simulink model "TX_Model"  (R2017a)
settings: Solver=VariableStepDiscrete  StartTime=0.0  StopTime=0.01  FixedStep=1/(PSF_SampPerSym*Rsymbol*2)  RelTol=1e-3  EnableMultiTasking=on
PreLoadFcn:
  | %Rates
  | BitRate=250e3;
  | ChipRate=2e6;
  | SymRate=ChipRate/2;
  | RX_ChipDelay=6;
  | 
  | 
  | %Pulse shaping filter
  | OS=32;
  | 
  | %Input Power
  | Pin=-12;
InitFcn:
  | x=linspace(0,1,OS);
  | weights=sin(pi*x);
libraries: dspmlti4 x1, commrandsrc2 x1, commseqgen2 x1, dspmathops x1, commdigbbndpm3 x1
settings Model: Creator=The MathWorks Inc.  LastModifiedBy=gzucchel
settings DataIOCC: LimitDataPoints=on  SaveFormat=Array  SignalLoggingSaveFormat=ModelDataLogs  SaveOutput=off  SignalLogging=off  DSMLogging=off  SaveTime=off
settings OptimizationCC: ExpressionDepthLimit=2147483647  LifeSpan=inf
settings DebuggingCC: UnderspecifiedInitializationDetection=Classic  MergeDetectMultiDrivingBlocksExec=none  SolverPrmCheckMsg=warning  FcnCallInpInsideContextMsg=warning  StateNameClashWarn=warning  SFUnexpectedBacktrackingDiag=warning  SFNoUnconditionalDefaultTransitionDiag=warning  SFExecutionAtInitializationDiag=none
settings HardwareCC: ProdBitPerPointer=32  ProdBitPerSizeT=32  ProdBitPerPtrDiffT=32  ProdLargestAtomicFloat=None  ProdIntDivRoundTo=Undefined  ProdEndianess=Unspecified  ProdWordSize=32  ProdHWDeviceType=32-bit Generic
settings ModelReferenceCC: PropagateSignalLabelsOutOfModel=off
settings GRTTargetCC: TargetLangStandard=C89/C90 (ANSI)  GeneratePreprocessorConditionals=Disable all  CombineOutputUpdateFcns=off  GRTInterface=on
settings ConfigComp: CovMetricSettings=dw  CovHtmlReporting=on  CovSaveCumulativeToWorkspaceVar=on  CovSaveSingleToWorkspaceVar=on  CovExternalEMLEnable=off  CovSFcnEnable=off
settings SimscapeCC: SimscapeNormalizeSystem=off  SimscapeNominalValues="[{\"value\":\"10\",\"unit\":\"V\"},{\"value\":\"1\",\"unit\":\"A\"},{\"value\":\"10\",\"unit\":\"N*m\"},{\"value\":\"10\",\"unit\":\"bar\"},{\"value\":\"100\",\"unit\":\"kJ/kg\"},{\"value\":\"1\",\"unit\":\"kW\"},{\"value\":\"300\",\"unit\":\"K\"},{\"value\":\"100\",\"unit\":\"cm^3/s\"},{\"value\":\"1\",\"unit\":\"kN\"},{\"value\":\"1\",\"unit\":\"g/cm^3\"},{\"value\":\"1\",\"unit\":\"l\"},{\"value\":\"1\",\"unit\":\"cm^2\"},{\"value\":\"60\",\"unit\":\"Hz\"}]"
settings ConfigurationSet: Description=SimMechanics 2G

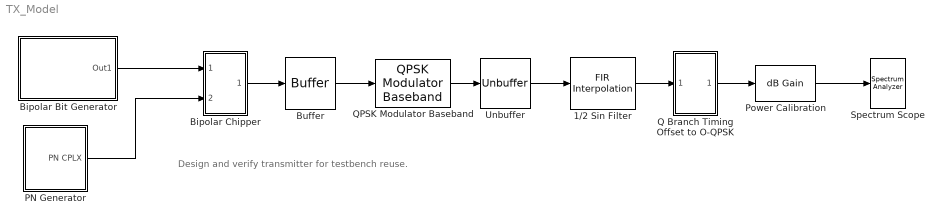
== system TX_Model ==
  note: Design and verify transmitter for testbench reuse.
  1/2 Sin Filter : dspmlti4/FIR Interpolation  FilterSource=Dialog parameters  h=weights  L=OS  FilterObject=Hm_firinterp  framing=Allow multirate processing  outputBufInitCond=0  roundingMode=Floor  overflowMode=off  firstCoeffDataTypeStr=Inherit: Same word length as input  firstCoeffMin=[]  firstCoeffMax=[]  firstCoeffLastDataTypeStr=Inherit: Same word length as input  outputDataTypeStr=Inherit: Same as accumulator  outputMin=[]  outputMax=[]  outputLastDataTypeStr=Inherit: Same as accumulator
      settings: SourceProductName=DSP System Toolbox
  Bipolar Chipper : Subsystem
  Bipolar Bit Generator : Subsystem
  Buffer : Buffer  N=2
  PN Generator : Subsystem
  Power Calibration : dspmathops/dB Gain  dB=Pin-26.7  intype=Amplitude
      settings: SourceProductName=DSP System Toolbox  SourceProductBaseCode=DS
  Q Branch Timing Offset to O-QPSK : Subsystem
  QPSK Modulator Baseband : commdigbbndpm3/QPSK Modulator Baseband  InType=Bit  Enc=Gray  Ph=pi/4  outDtype=double  outWordLen=16  outUDDataType=sfix(16)  outFracLenMode=Best precision  outFracLen=15  outDataTypeStr=double  outLastDataTypeStr=double
  Spectrum Scope : SpectrumAnalyzer
  Unbuffer : Unbuffer
  wires:
  QPSK Modulator Baseband/1 -> Unbuffer/1
  1/2 Sin Filter/1 -> Q Branch Timing Offset to O-QPSK/1(In1)
  Q Branch Timing Offset to O-QPSK/1(Out1) -> Power Calibration/1
  PN Generator/1(PN CPLX) -> Bipolar Chipper/2(In2)
  Bipolar Bit Generator/1(Out1) -> Bipolar Chipper/1(In1)
  Bipolar Chipper/1(Out1) -> Buffer/1
  Buffer/1 -> QPSK Modulator Baseband/1
  Unbuffer/1 -> 1/2 Sin Filter/1
  Power Calibration/1 -> Spectrum Scope/1

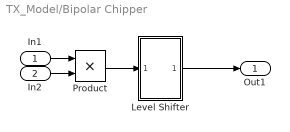
== system TX_Model/Bipolar Chipper ==
  In1 : Inport
  In2 : Inport  Port=2
  Level Shifter : Subsystem
  Product : Product  RndMeth=Zero
  Out1 : Outport
  wires:
  In2/1 -> Product/2
  Level Shifter/1(Out1) -> Out1/1
  In1/1 -> Product/1
  Product/1 -> Level Shifter/1(In1)

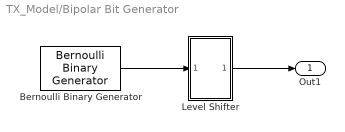
== system TX_Model/Bipolar Bit Generator ==
  Bernoulli Binary Generator : commrandsrc2/Bernoulli Binary Generator  P=0.5  seed=61  Ts=1/BitRate  frameBased=off  sampPerFrame=1  orient=off  outDataType=double
  Level Shifter : Subsystem
  Out1 : Outport
  wires:
  Level Shifter/1(Out1) -> Out1/1
  Bernoulli Binary Generator/1 -> Level Shifter/1(In1)

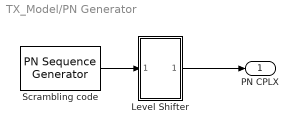
== system TX_Model/PN Generator ==
  Level Shifter : Subsystem
  Scrambling code : commseqgen2/PN Sequence Generator  poly=[0 -7 -10]  ini_sta=[1 0 0 0 0 0 0 0 0 0]  outBitMaskSource=Dialog parameter  shift=0  outVarSiz=off  maxOutSizeMode=Dialog parameter  maxOutSize=[10 1]  Ts=1/ChipRate  frameBased=off  sampPerFrame=1  reset=off  bitPackedOutputs=off  outDataType=double  numPackedBits=8  bitPackDataSigned=off  bitPackedOutDType=double
  PN CPLX : Outport
  wires:
  Level Shifter/1(Out1) -> PN CPLX/1
  Scrambling code/1 -> Level Shifter/1(In1)

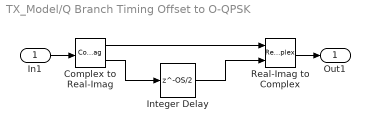
== system TX_Model/Q Branch Timing Offset to O-QPSK ==
  In1 : Inport
  Complex to Real-Imag : ComplexToRealImag
  Integer Delay : Delay  DelayLength=OS/2
  Real-Imag to Complex : RealImagToComplex
  Out1 : Outport
  wires:
  Real-Imag to Complex/1 -> Out1/1
  In1/1 -> Complex to Real-Imag/1
  Complex to Real-Imag/1 -> Real-Imag to Complex/1
  Integer Delay/1 -> Real-Imag to Complex/2
  Complex to Real-Imag/2 -> Integer Delay/1

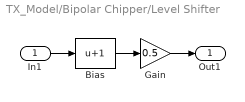
== system TX_Model/Bipolar Chipper/Level Shifter ==
  In1 : Inport
  Bias : Bias  Bias=1
  Gain : Gain  Gain=0.5
  Out1 : Outport
  wires:
  Gain/1 -> Out1/1
  In1/1 -> Bias/1
  Bias/1 -> Gain/1

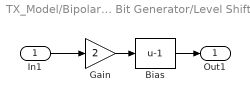
== system TX_Model/Bipolar Bit Generator/Level Shifter ==
  In1 : Inport
  Bias : Bias  Bias=-1
  Gain : Gain  Gain=2
  Out1 : Outport
  wires:
  Bias/1 -> Out1/1
  In1/1 -> Gain/1
  Gain/1 -> Bias/1

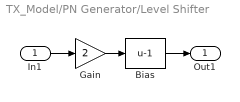
== system TX_Model/PN Generator/Level Shifter ==
  In1 : Inport
  Bias : Bias  Bias=-1
  Gain : Gain  Gain=2
  Out1 : Outport
  wires:
  In1/1 -> Gain/1
  Bias/1 -> Out1/1
  Gain/1 -> Bias/1
